simulink model "lab2_star_star"  (R2015a)
settings: Solver=ode45  StartTime=0.0  StopTime=1  RelTol=1e-3
libraries: powerlib x11
settings Model: Creator=DHARMIK  LastModifiedBy=DHARMIK

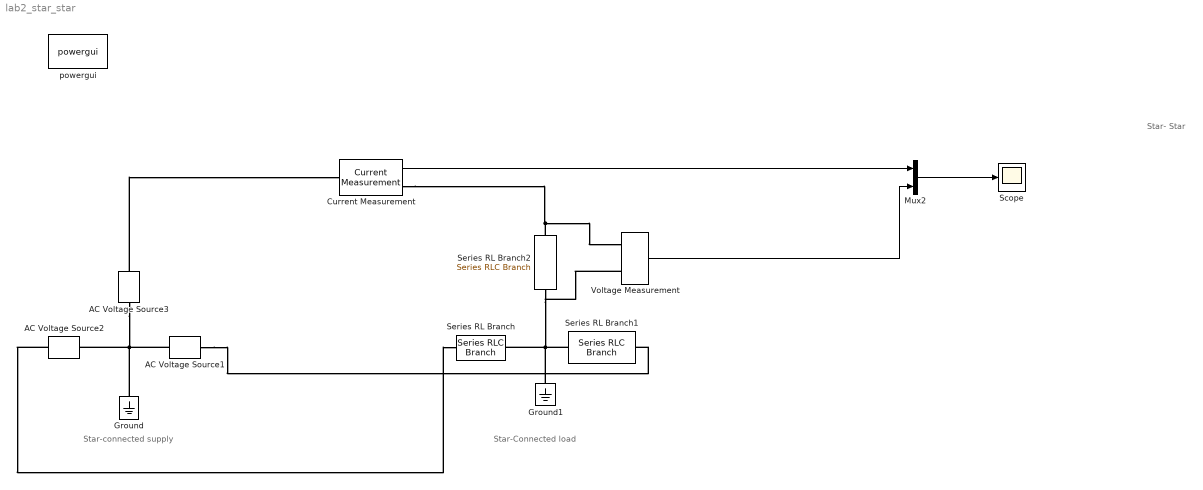
== system lab2_star_star ==
  note: Star- Star
  note: Star-Connected load
  note: Star-connected supply
  AC Voltage Source1 : powerlib/Electrical Sources/AC Voltage Source  Amplitude=187.79  Phase=120  Frequency=50  SampleTime=0  Measurements=None
  AC Voltage Source2 : powerlib/Electrical Sources/AC Voltage Source  Amplitude=187.79  Phase=240  Frequency=50  SampleTime=0  Measurements=None
  AC Voltage Source3 : powerlib/Electrical Sources/AC Voltage Source  Amplitude=187.79  Phase=0  Frequency=50  SampleTime=0  Measurements=None
  Current Measurement : powerlib/Measurements/Current Measurement  PhasorSimulation=off  OutputType=Complex  PSBequivalent=0
  Ground : powerlib/Elements/Ground  LConnTagsString=a
  Ground1 : powerlib/Elements/Ground  LConnTagsString=a
  Mux2 : Mux  Inputs=2
  Scope : Scope
      settings: ShowLegends=on  YMin=1373.1  YMax=3560.58  SaveName=ScopeData2
  Series RL Branch : powerlib/Elements/Series RLC Branch  LConnTagsString=__new0  RConnTagsString=__new0  BranchType=RL  Resistance=4.28  Inductance=0.0066017  SetiL0=off  InitialCurrent=0  Capacitance=0  Setx0=off  InitialVoltage=0  Measurements=None
  Series RL Branch1 : powerlib/Elements/Series RLC Branch  LConnTagsString=__new0  RConnTagsString=__new0  BranchType=RL  Resistance=4.28  Inductance=0.0066017  SetiL0=off  InitialCurrent=0  Capacitance=0  Setx0=off  InitialVoltage=0  Measurements=None
  Series RL Branch2 : powerlib/Elements/Series RLC Branch  LConnTagsString=__new0  RConnTagsString=__new0  BranchType=RL  Resistance=4.28  Inductance=0.0066017  SetiL0=off  InitialCurrent=0  Capacitance=0  Setx0=off  InitialVoltage=0  Measurements=None
  Voltage Measurement : powerlib/Measurements/Voltage Measurement  PhasorSimulation=off  OutputType=Complex  PSBequivalent=0
  powergui : powerlib/powergui  Priority=1  SimulationMode=Discrete  SolverType=Tustin/Backward Euler (TBE)  SampleTime=50e-6  frequency=60  SPID=off  DisableSnubberDevices=off  DisableRonSwitches=off  DisableVfSwitches=off  SwTol=0  DisplayEquations=off  Interpol=off  methode=off  Ts=100  FunctionMessages=off  echomessages=off  HookPort=off  EnableUseOfTLC=off  x0status=blocks  frequencyindice=50  Pbase=100e6  ErrMax=1e-4  Iterations=50  UnitsV=kV  UnitsW=MW  buscounter=0  RestoreLinks=warning  ResistiveCurrentMeasurement=off  Frange=[0:2:500]  Ylog=off  Xlog=on  ShowGrid=off  save=off  variable=ZData  structure=0  ZoomFFT=off  StartTime=0.0  cycles=1  DisplayStyle=1  fundamental=60  FreqAxis=off  MaxFrequency=1000  frequencyindicesteady=1  RmsSteady=1  display=off
  wires:
  Mux2/1 -> Scope/1
  Voltage Measurement/1 -> Mux2/2
  Current Measurement/1 -> Mux2/1
  connections:
  Series RL Branch2/RConn1 -- Voltage Measurement/LConn2 -- Series RL Branch1/RConn1 -- Series RL Branch/LConn1 -- Ground1/LConn1
  AC Voltage Source3/LConn1 -- AC Voltage Source1/LConn1 -- Ground/LConn1 -- AC Voltage Source2/LConn1
  AC Voltage Source2/RConn1 -- Series RL Branch/RConn1
  Series RL Branch2/LConn1 -- Voltage Measurement/LConn1 -- Current Measurement/RConn1
  AC Voltage Source1/RConn1 -- Series RL Branch1/LConn1
  AC Voltage Source3/RConn1 -- Current Measurement/LConn1
